simulink model "BEX7_CANOpen_Torque_Speed_Position_Control_Generic_2022b"  (R2022b)
settings: Solver=VariableStepAuto  StartTime=0.0  StopTime=inf  RelTol=1e-3
(part 2 of 2)

== system BEX7_CANOpen_Torque_Speed_Position_Control_Generic_2022b/Tx/Subsystem2/Enabled Subsystem1 ==
  CurrentLimit : Inport
  Enable : EnablePort
  Constant6 : Constant  Value=0  OutDataTypeStr=uint8
  SetCurrentLimit : Subsystem
  Result : Outport
  Error : Outport  Port=2
  wires:
  Constant6/1 -> SetCurrentLimit/1(Address)
  CurrentLimit/1 -> SetCurrentLimit/2(Value)
  SetCurrentLimit/2(Error) -> Error/1
  SetCurrentLimit/1(Result) -> Result/1

== system BEX7_CANOpen_Torque_Speed_Position_Control_Generic_2022b/Tx/Subsystem2/Enabled Subsystem2 ==
  Number of Poles : Inport
  Enable : EnablePort
  Constant6 : Constant  Value=0  OutDataTypeStr=uint8
  SetMotorPoleCounts : Subsystem
  Result : Outport
  Error : Outport  Port=2
  wires:
  Number of Poles/1 -> SetMotorPoleCounts/2(Value)
  Constant6/1 -> SetMotorPoleCounts/1(Address)
  SetMotorPoleCounts/2(Error) -> Error/1
  SetMotorPoleCounts/1(Result) -> Result/1

== system BEX7_CANOpen_Torque_Speed_Position_Control_Generic_2022b/Tx/Subsystem2/Enabled Subsystem3 ==
  EncoderLines : Inport
  Enable : EnablePort
  Constant6 : Constant  Value=0  OutDataTypeStr=uint8
  SetEncoderLines : Subsystem
  Result : Outport
  Error : Outport  Port=2
  wires:
  Constant6/1 -> SetEncoderLines/1(Address)
  EncoderLines/1 -> SetEncoderLines/2(Value)
  SetEncoderLines/2(Error) -> Error/1
  SetEncoderLines/1(Result) -> Result/1

== system BEX7_CANOpen_Torque_Speed_Position_Control_Generic_2022b/Tx/Subsystem2/Enabled Subsystem4 ==
  C.C.W Offset : Inport
  Enable : EnablePort
  Constant6 : Constant  Value=0  OutDataTypeStr=uint8
  SetEncoderHallCcwOffset : Subsystem
  Result : Outport
  Error : Outport  Port=2
  wires:
  C.C.W Offset/1 -> SetEncoderHallCcwOffset/2(Value)
  Constant6/1 -> SetEncoderHallCcwOffset/1(Address)
  SetEncoderHallCcwOffset/2(Error) -> Error/1
  SetEncoderHallCcwOffset/1(Result) -> Result/1

== system BEX7_CANOpen_Torque_Speed_Position_Control_Generic_2022b/Tx/Subsystem2/Enabled Subsystem5 ==
  C.W Offset : Inport
  Enable : EnablePort
  Constant6 : Constant  Value=0  OutDataTypeStr=uint8
  SetEncoderHallCwOffset : Subsystem
  Result : Outport
  Error : Outport  Port=2
  wires:
  Constant6/1 -> SetEncoderHallCwOffset/1(Address)
  C.W Offset/1 -> SetEncoderHallCwOffset/2(Value)
  SetEncoderHallCwOffset/2(Error) -> Error/1
  SetEncoderHallCwOffset/1(Result) -> Result/1

== system BEX7_CANOpen_Torque_Speed_Position_Control_Generic_2022b/Tx/Subsystem2/Enabled Subsystem6 ==
  SpeedLimit : Inport
  Enable : EnablePort
  Constant6 : Constant  Value=0  OutDataTypeStr=uint8
  SetSpeedLimit : Subsystem
  Result : Outport
  Error : Outport  Port=2
  wires:
  SpeedLimit/1 -> SetSpeedLimit/2(Value)
  Constant6/1 -> SetSpeedLimit/1(Address)
  SetSpeedLimit/2(Error) -> Error/1
  SetSpeedLimit/1(Result) -> Result/1

== system BEX7_CANOpen_Torque_Speed_Position_Control_Generic_2022b/Tx/Subsystem2/Enabled Subsystem7 ==
  ControlMode : Inport
  Enable : EnablePort
  Constant6 : Constant  Value=0  OutDataTypeStr=uint8
  SetControlMode : Subsystem
  Result : Outport
  Error : Outport  Port=2
  wires:
  Constant6/1 -> SetControlMode/1(Address)
  ControlMode/1 -> SetControlMode/2(Value)
  SetControlMode/2(Error) -> Error/1
  SetControlMode/1(Result) -> Result/1

== system BEX7_CANOpen_Torque_Speed_Position_Control_Generic_2022b/Tx/Subsystem2/Enabled Subsystem8 ==
  MotorType : Inport
  Enable : EnablePort
  Constant6 : Constant  Value=0  OutDataTypeStr=uint8
  SetMotorType : Subsystem
  Result : Outport
  Error : Outport  Port=2
  wires:
  MotorType/1 -> SetMotorType/2(Value)
  Constant6/1 -> SetMotorType/1(Address)
  SetMotorType/2(Error) -> Error/1
  SetMotorType/1(Result) -> Result/1

== system BEX7_CANOpen_Torque_Speed_Position_Control_Generic_2022b/Tx/Subsystem2/Enabled Subsystem9 ==
  FeedbackMode : Inport
  Enable : EnablePort
  Constant6 : Constant  Value=0  OutDataTypeStr=uint8
  SetFeedBackControlMode : Subsystem
  Result : Outport
  Error : Outport  Port=2
  wires:
  Constant6/1 -> SetFeedBackControlMode/1(Address)
  FeedbackMode/1 -> SetFeedBackControlMode/2(Value)
  SetFeedBackControlMode/2(Error) -> Error/1
  SetFeedBackControlMode/1(Result) -> Result/1

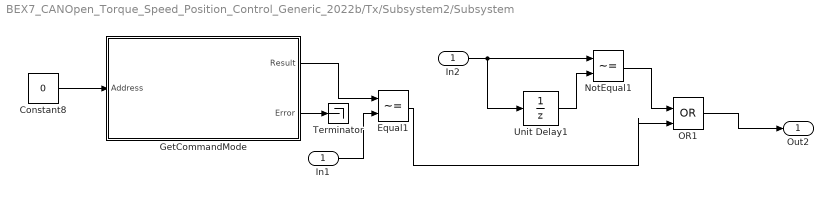
== system BEX7_CANOpen_Torque_Speed_Position_Control_Generic_2022b/Tx/Subsystem2/Subsystem ==
  In1 : Inport
  Constant8 : Constant  Value=0  OutDataTypeStr=uint8
  Equal1 : RelationalOperator  Operator=~=  OutDataTypeStr=boolean  RndMeth=Simplest  InputSameDT=off
  GetCommandMode : Subsystem
  In2 : InportShadow
  NotEqual1 : RelationalOperator  Operator=~=  OutDataTypeStr=boolean  RndMeth=Simplest  InputSameDT=off
  OR1 : Logic  Operator=OR  IconShape=distinctive  AllPortsSameDT=off  OutDataTypeStr=boolean
  Terminator : Terminator
  Unit Delay1 : UnitDelay  InitialCondition=2.1651  SampleTime=-1  HasFrameUpgradeWarning=on
  Out2 : Outport
  wires:
  In2/1 -> Unit Delay1/1, NotEqual1/1
  In1/1 -> Equal1/2
  GetCommandMode/2(Error) -> Terminator/1
  Equal1/1 -> OR1/2
  NotEqual1/1 -> OR1/1
  GetCommandMode/1(Result) -> Equal1/1
  Constant8/1 -> GetCommandMode/1(Address)
  Unit Delay1/1 -> NotEqual1/2
  OR1/1 -> Out2/1

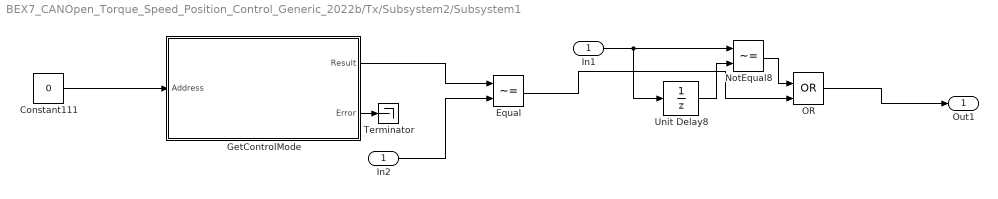
== system BEX7_CANOpen_Torque_Speed_Position_Control_Generic_2022b/Tx/Subsystem2/Subsystem1 ==
  In1 : Inport
  Constant111 : Constant  Value=0  OutDataTypeStr=uint8
  Equal : RelationalOperator  Operator=~=  OutDataTypeStr=boolean  RndMeth=Simplest  InputSameDT=off
  GetControlMode : Subsystem
  In2 : InportShadow
  NotEqual8 : RelationalOperator  Operator=~=  OutDataTypeStr=boolean  RndMeth=Simplest  InputSameDT=off
  OR : Logic  Operator=OR  IconShape=distinctive  AllPortsSameDT=off  OutDataTypeStr=boolean
  Terminator : Terminator
  Unit Delay8 : UnitDelay  InitialCondition=2.1651  SampleTime=-1  HasFrameUpgradeWarning=on
  Out1 : Outport
  wires:
  OR/1 -> Out1/1
  Unit Delay8/1 -> NotEqual8/2
  In1/1 -> Unit Delay8/1, NotEqual8/1
  Equal/1 -> OR/2
  GetControlMode/1(Result) -> Equal/1
  NotEqual8/1 -> OR/1
  GetControlMode/2(Error) -> Terminator/1
  Constant111/1 -> GetControlMode/1(Address)
  In2/1 -> Equal/2

== system BEX7_CANOpen_Torque_Speed_Position_Control_Generic_2022b/Tx/Subsystem1/Enabled Subsystem/SetTorqueReferenceIq ==
  Address : Inport  OutDataTypeStr=uint8  LockScale=on
  Value : Inport  Port=2  OutDataTypeStr=single  LockScale=on
  Display12 : Display
      settings: Format=decimal (Stored Integer)
  Display13 : Display
      settings: Format=decimal (Stored Integer)
  S-Function Builder4 : S-Function  Priority=2  FunctionName=SetTorqueReferenceIq  SFunctionModules=SetTorqueReferenceIq_wrapper  SFunctionDeploymentMode=off  EnableBusSupport=off  mask(S-Function Builder){}
      mask help: Simulink:masks:SFunctionBuilder_MD
      mask init: same as BEX7_CANOpen_Torque_Speed_Position_Control_Generic_2022b/Subsystem1/Subsystem/S-Function Builder1
      settings: CopyFcn=set_param(gcbh,'LinkStatus','none')  OpenFcn=sfunctionwizard(gcbh)
      mask Display: plot(val(:,1),val(:,2)),disp(sys),port_label('input',1,'Address'),port_label('input',2,'Value'),port_label('output',1,'Result'),port_label('output',2,'Error')
  Result : Outport  OutDataTypeStr=boolean
  Error : Outport  Port=2  OutDataTypeStr=int32
  wires:
  Address/1 -> S-Function Builder4/1
  S-Function Builder4/2 -> Error/1, Display13/1
  S-Function Builder4/1 -> Result/1, Display12/1
  Value/1 -> S-Function Builder4/2

== system BEX7_CANOpen_Torque_Speed_Position_Control_Generic_2022b/Tx/Subsystem1/Enabled Subsystem1/SpeedRef ==
  Address : Inport
  Value : Inport  Port=2
  Display16 : Display
      settings: Format=decimal (Stored Integer)
  Display17 : Display
      settings: Format=decimal (Stored Integer)
  S-Function Builder8 : S-Function  Priority=2  FunctionName=SetSpeedReference  SFunctionModules=SetSpeedReference_wrapper  SFunctionDeploymentMode=off  EnableBusSupport=off  mask(S-Function Builder){}
      mask help: Simulink:masks:SFunctionBuilder_MD
      mask init: same as BEX7_CANOpen_Torque_Speed_Position_Control_Generic_2022b/Subsystem1/Subsystem/S-Function Builder1
      settings: CopyFcn=set_param(gcbh,'LinkStatus','none')  OpenFcn=sfunctionwizard(gcbh)
      mask Display:
      | plot(val(:,1),val(:,2))
      | disp(sys)
      | port_label('input',1,'Address')
      | port_label('input',2,'Value')
      | port_label('output',1,'Result')
      | port_label('output',2,'Error')
  Result : Outport
  Error : Outport  Port=2
  wires:
  Address/1 -> S-Function Builder8/1
  S-Function Builder8/1 -> Result/1, Display16/1
  S-Function Builder8/2 -> Error/1, Display17/1
  Value/1 -> S-Function Builder8/2

== system BEX7_CANOpen_Torque_Speed_Position_Control_Generic_2022b/Tx/Subsystem1/Enabled Subsystem10/EmergencyStop1 ==
  note: Error
  Address : Inport
  Display22 : Display
      settings: Format=decimal (Stored Integer)
  Display23 : Display
      settings: Format=decimal (Stored Integer)
  S-Function Builder11 : S-Function  Priority=2  FunctionName=EmergencyStop  SFunctionModules=EmergencyStop_wrapper  SFunctionDeploymentMode=off  EnableBusSupport=off  mask(S-Function Builder){}
      mask help: Simulink:masks:SFunctionBuilder_MD
      mask init: same as BEX7_CANOpen_Torque_Speed_Position_Control_Generic_2022b/Subsystem1/Subsystem/S-Function Builder1
      settings: CopyFcn=set_param(gcbh,'LinkStatus','none')  OpenFcn=sfunctionwizard(gcbh)
      mask Display:
      | plot(val(:,1),val(:,2))
      | disp(sys)
      | port_label('input',1,'Address')
      | port_label('output',1,'Result')
      | port_label('output',2,'Error')
  Result : Outport
  Error : Outport  Port=2
  wires:
  S-Function Builder11/2 -> Error/1, Display23/1
  S-Function Builder11/1 -> Result/1, Display22/1
  Address/1 -> S-Function Builder11/1

== system BEX7_CANOpen_Torque_Speed_Position_Control_Generic_2022b/Tx/Subsystem1/Enabled Subsystem2/SetPositionRef ==
  Address : Inport
  Value : Inport  Port=2
  S-Function Builder30 : S-Function  Priority=2  FunctionName=SetPositionReference  SFunctionModules=SetPositionReference_wrapper  SFunctionDeploymentMode=off  EnableBusSupport=off  mask(S-Function Builder){}
      mask help: Simulink:masks:SFunctionBuilder_MD
      mask init: same as BEX7_CANOpen_Torque_Speed_Position_Control_Generic_2022b/Subsystem1/Subsystem/S-Function Builder1
      settings: CopyFcn=set_param(gcbh,'LinkStatus','none')  OpenFcn=sfunctionwizard(gcbh)
      mask Display:
      | plot(val(:,1),val(:,2))
      | disp(sys)
      | port_label('input',1,'Address')
      | port_label('input',2,'Value')
      | port_label('output',1,'Result')
      | port_label('output',2,'Error')
  Result : Outport
  Error : Outport  Port=2
  wires:
  S-Function Builder30/1 -> Result/1
  S-Function Builder30/2 -> Error/1
  Value/1 -> S-Function Builder30/2
  Address/1 -> S-Function Builder30/1

== system BEX7_CANOpen_Torque_Speed_Position_Control_Generic_2022b/Tx/Subsystem1/Enabled Subsystem3/SetMotorDirection ==
  Address : Inport
  Value : Inport  Port=2
  S-Function Builder15 : S-Function  Priority=2  FunctionName=SetMotorDirection  SFunctionModules=SetMotorDirection_wrapper  SFunctionDeploymentMode=off  EnableBusSupport=off  mask(S-Function Builder){}
      mask help: Simulink:masks:SFunctionBuilder_MD
      mask init: same as BEX7_CANOpen_Torque_Speed_Position_Control_Generic_2022b/Subsystem1/Subsystem/S-Function Builder1
      settings: CopyFcn=set_param(gcbh,'LinkStatus','none')  OpenFcn=sfunctionwizard(gcbh)
      mask Display: plot(val(:,1),val(:,2)),disp(sys),port_label('input',1,'Address'),port_label('input',2,'Value'),port_label('output',1,'Result'),port_label('output',2,'Error')
  Result : Outport
  Error : Outport  Port=2
  wires:
  S-Function Builder15/2 -> Error/1
  Value/1 -> S-Function Builder15/2
  S-Function Builder15/1 -> Result/1
  Address/1 -> S-Function Builder15/1

== system BEX7_CANOpen_Torque_Speed_Position_Control_Generic_2022b/Tx/Subsystem1/Enabled Subsystem4/SetSpeed Kp ==
  Address : Inport
  Value : Inport  Port=2
  Display26 : Display
      settings: Format=decimal (Stored Integer)
  Display27 : Display
      settings: Format=decimal (Stored Integer)
  S-Function Builder13 : S-Function  Priority=2  FunctionName=SetSpeedControllerKp  SFunctionModules=SetSpeedControllerKp_wrapper  SFunctionDeploymentMode=off  EnableBusSupport=off  mask(S-Function Builder){}
      mask help: Simulink:masks:SFunctionBuilder_MD
      mask init: same as BEX7_CANOpen_Torque_Speed_Position_Control_Generic_2022b/Subsystem1/Subsystem/S-Function Builder1
      settings: CopyFcn=set_param(gcbh,'LinkStatus','none')  OpenFcn=sfunctionwizard(gcbh)
      mask Display:
      | plot(val(:,1),val(:,2))
      | disp(sys)
      | port_label('input',1,'Address')
      | port_label('input',2,'Value')
      | port_label('output',1,'Result')
      | port_label('output',2,'Error')
  Result : Outport
  Error : Outport  Port=2
  wires:
  S-Function Builder13/1 -> Result/1, Display26/1
  S-Function Builder13/2 -> Error/1, Display27/1
  Address/1 -> S-Function Builder13/1
  Value/1 -> S-Function Builder13/2

== system BEX7_CANOpen_Torque_Speed_Position_Control_Generic_2022b/Tx/Subsystem1/Enabled Subsystem5/SetSpeed Ki ==
  Address : Inport
  Value : Inport  Port=2
  Display28 : Display
      settings: Format=decimal (Stored Integer)
  Display29 : Display
      settings: Format=decimal (Stored Integer)
  S-Function Builder14 : S-Function  Priority=2  FunctionName=SetSpeedControllerKi  SFunctionModules=SetSpeedControllerKi_wrapper  SFunctionDeploymentMode=off  EnableBusSupport=off  mask(S-Function Builder){}
      mask help: Simulink:masks:SFunctionBuilder_MD
      mask init: same as BEX7_CANOpen_Torque_Speed_Position_Control_Generic_2022b/Subsystem1/Subsystem/S-Function Builder1
      settings: CopyFcn=set_param(gcbh,'LinkStatus','none')  OpenFcn=sfunctionwizard(gcbh)
      mask Display:
      | plot(val(:,1),val(:,2))
      | disp(sys)
      | port_label('input',1,'Address')
      | port_label('input',2,'Value')
      | port_label('output',1,'Result')
      | port_label('output',2,'Error')
  Result : Outport
  Error : Outport  Port=2
  wires:
  S-Function Builder14/1 -> Result/1, Display28/1
  Value/1 -> S-Function Builder14/2
  S-Function Builder14/2 -> Error/1, Display29/1
  Address/1 -> S-Function Builder14/1

== system BEX7_CANOpen_Torque_Speed_Position_Control_Generic_2022b/Tx/Subsystem1/Enabled Subsystem6/SetPositionControllerKp ==
  Address : Inport
  Value : Inport  Port=2
  Display62 : Display
      settings: Format=decimal (Stored Integer)
  Display63 : Display
      settings: Format=decimal (Stored Integer)
  S-Function Builder31 : S-Function  Priority=2  FunctionName=SetPositionControllerKp  SFunctionModules=SetPositionControllerKp_wrapper  SFunctionDeploymentMode=off  EnableBusSupport=off  mask(S-Function Builder){}
      mask help: Simulink:masks:SFunctionBuilder_MD
      mask init: same as BEX7_CANOpen_Torque_Speed_Position_Control_Generic_2022b/Subsystem1/Subsystem/S-Function Builder1
      settings: CopyFcn=set_param(gcbh,'LinkStatus','none')  OpenFcn=sfunctionwizard(gcbh)
      mask Display:
      | plot(val(:,1),val(:,2))
      | disp(sys)
      | port_label('input',1,'Address')
      | port_label('input',2,'Value')
      | port_label('output',1,'Result')
      | port_label('output',2,'Error')
  Result : Outport
  Error : Outport  Port=2
  wires:
  S-Function Builder31/2 -> Error/1, Display63/1
  Value/1 -> S-Function Builder31/2
  Address/1 -> S-Function Builder31/1
  S-Function Builder31/1 -> Result/1, Display62/1

== system BEX7_CANOpen_Torque_Speed_Position_Control_Generic_2022b/Tx/Subsystem1/Enabled Subsystem7/SetPositionControllerKi ==
  Address : Inport
  Value : Inport  Port=2
  Display64 : Display
      settings: Format=decimal (Stored Integer)
  Display65 : Display
      settings: Format=decimal (Stored Integer)
  S-Function Builder32 : S-Function  Priority=2  FunctionName=SetPositionControllerKi  SFunctionModules=SetPositionControllerKi_wrapper  SFunctionDeploymentMode=off  EnableBusSupport=off  mask(S-Function Builder){}
      mask help: Simulink:masks:SFunctionBuilder_MD
      mask init: same as BEX7_CANOpen_Torque_Speed_Position_Control_Generic_2022b/Subsystem1/Subsystem/S-Function Builder1
      settings: CopyFcn=set_param(gcbh,'LinkStatus','none')  OpenFcn=sfunctionwizard(gcbh)
      mask Display:
      | plot(val(:,1),val(:,2))
      | disp(sys)
      | port_label('input',1,'Address')
      | port_label('input',2,'Value')
      | port_label('output',1,'Result')
      | port_label('output',2,'Error')
  Result : Outport
  Error : Outport  Port=2
  wires:
  S-Function Builder32/1 -> Result/1, Display64/1
  Value/1 -> S-Function Builder32/2
  S-Function Builder32/2 -> Error/1, Display65/1
  Address/1 -> S-Function Builder32/1

== system BEX7_CANOpen_Torque_Speed_Position_Control_Generic_2022b/Tx/Subsystem1/Enabled Subsystem8/SetCurrentControlKp ==
  Address : Inport
  Value : Inport  Port=2
  Display52 : Display
      settings: Format=decimal (Stored Integer)
  Display53 : Display
      settings: Format=decimal (Stored Integer)
  S-Function Builder26 : S-Function  Priority=2  FunctionName=SetCurrentControllerKp  SFunctionModules=SetCurrentControllerKp_wrapper  SFunctionDeploymentMode=off  EnableBusSupport=off  mask(S-Function Builder){}
      mask help: Simulink:masks:SFunctionBuilder_MD
      mask init: same as BEX7_CANOpen_Torque_Speed_Position_Control_Generic_2022b/Subsystem1/Subsystem/S-Function Builder1
      settings: CopyFcn=set_param(gcbh,'LinkStatus','none')  OpenFcn=sfunctionwizard(gcbh)
      mask Display:
      | plot(val(:,1),val(:,2))
      | disp(sys)
      | port_label('input',1,'Address')
      | port_label('input',2,'Value')
      | port_label('output',1,'Result')
      | port_label('output',2,'Error')
  Result : Outport
  Error : Outport  Port=2
  wires:
  Value/1 -> S-Function Builder26/2
  S-Function Builder26/1 -> Result/1, Display52/1
  Address/1 -> S-Function Builder26/1
  S-Function Builder26/2 -> Error/1, Display53/1

== system BEX7_CANOpen_Torque_Speed_Position_Control_Generic_2022b/Tx/Subsystem1/Enabled Subsystem9/SetCurrentControlKi ==
  Address : Inport
  Value : Inport  Port=2
  Display54 : Display
      settings: Format=decimal (Stored Integer)
  Display55 : Display
      settings: Format=decimal (Stored Integer)
  S-Function Builder27 : S-Function  Priority=2  FunctionName=SetCurrentControllerKi  SFunctionModules=SetCurrentControllerKi_wrapper  SFunctionDeploymentMode=off  EnableBusSupport=off  mask(S-Function Builder){}
      mask help: Simulink:masks:SFunctionBuilder_MD
      mask init: same as BEX7_CANOpen_Torque_Speed_Position_Control_Generic_2022b/Subsystem1/Subsystem/S-Function Builder1
      settings: CopyFcn=set_param(gcbh,'LinkStatus','none')  OpenFcn=sfunctionwizard(gcbh)
      mask Display:
      | plot(val(:,1),val(:,2))
      | disp(sys)
      | port_label('input',1,'Address')
      | port_label('input',2,'Value')
      | port_label('output',1,'Result')
      | port_label('output',2,'Error')
  Result : Outport
  Error : Outport  Port=2
  wires:
  Value/1 -> S-Function Builder27/2
  S-Function Builder27/1 -> Result/1, Display54/1
  S-Function Builder27/2 -> Error/1, Display55/1
  Address/1 -> S-Function Builder27/1

== system BEX7_CANOpen_Torque_Speed_Position_Control_Generic_2022b/Tx/Subsystem1/Subsystem/GetMotorDirection ==
  Address : Inport
  S-Function Builder82 : S-Function  Priority=3  FunctionName=GetMotorDirection  SFunctionModules=GetMotorDirection_wrapper  SFunctionDeploymentMode=off  EnableBusSupport=off  mask(S-Function Builder){}
      mask help: Simulink:masks:SFunctionBuilder_MD
      mask init: same as BEX7_CANOpen_Torque_Speed_Position_Control_Generic_2022b/Subsystem1/Subsystem/S-Function Builder1
      settings: CopyFcn=set_param(gcbh,'LinkStatus','none')  OpenFcn=sfunctionwizard(gcbh)
      mask Display:
      | plot(val(:,1),val(:,2))
      | disp(sys)
      | port_label('input',1,'Address')
      | port_label('output',1,'Result')
      | port_label('output',2,'Error')
  Result : Outport
  Error : Outport  Port=2
  wires:
  S-Function Builder82/2 -> Error/1
  S-Function Builder82/1 -> Result/1
  Address/1 -> S-Function Builder82/1

== system BEX7_CANOpen_Torque_Speed_Position_Control_Generic_2022b/Tx/Subsystem2/Enabled Subsystem/SetCommandMode ==
  Address : Inport  OutDataTypeStr=uint8  LockScale=on
  Value : Inport  Port=2  OutDataTypeStr=boolean  LockScale=on
  S-Function Builder2 : S-Function  Priority=2  FunctionName=SetCommandMode  SFunctionModules=SetCommandMode_wrapper  SFunctionDeploymentMode=off  EnableBusSupport=off  mask(S-Function Builder){}
      mask help: Simulink:masks:SFunctionBuilder_MD
      mask init: same as BEX7_CANOpen_Torque_Speed_Position_Control_Generic_2022b/Subsystem1/Subsystem/S-Function Builder1
      settings: CopyFcn=set_param(gcbh,'LinkStatus','none')  OpenFcn=sfunctionwizard(gcbh)
      mask Display: plot(val(:,1),val(:,2)),disp(sys),port_label('input',1,'Address'),port_label('input',2,'Value'),port_label('output',1,'Result'),port_label('output',2,'Error')
  Result : Outport  OutDataTypeStr=boolean
  Error : Outport  Port=2
  wires:
  S-Function Builder2/1 -> Result/1
  S-Function Builder2/2 -> Error/1
  Address/1 -> S-Function Builder2/1
  Value/1 -> S-Function Builder2/2

== system BEX7_CANOpen_Torque_Speed_Position_Control_Generic_2022b/Tx/Subsystem2/Enabled Subsystem1/SetCurrentLimit ==
  Address : Inport  Tag=Address  LockScale=on
  Value : Inport  Port=2  LockScale=on
  Display1 : Display
      settings: Format=decimal (Stored Integer)
  Display10 : Display
      settings: Format=decimal (Stored Integer)
  S-Function Builder : S-Function  Priority=2  FunctionName=SetCurrentLimit  SFunctionModules=SetCurrentLimit_wrapper  SFunctionDeploymentMode=off  EnableBusSupport=off  mask(S-Function Builder){}
      mask help: Simulink:masks:SFunctionBuilder_MD
      mask init: same as BEX7_CANOpen_Torque_Speed_Position_Control_Generic_2022b/Subsystem1/Subsystem/S-Function Builder1
      settings: CopyFcn=set_param(gcbh,'LinkStatus','none')  OpenFcn=sfunctionwizard(gcbh)
      mask Display: plot(val(:,1),val(:,2)),disp(sys),port_label('input',1,'Address'),port_label('input',2,'Value'),port_label('output',1,'Result'),port_label('output',2,'Error')
  Result : Outport  OutDataTypeStr=boolean
  Error : Outport  Port=2  OutDataTypeStr=int32
  wires:
  Value/1 -> S-Function Builder/2
  S-Function Builder/2 -> Error/1, Display10/1
  S-Function Builder/1 -> Result/1, Display1/1
  Address/1 -> S-Function Builder/1

== system BEX7_CANOpen_Torque_Speed_Position_Control_Generic_2022b/Tx/Subsystem2/Enabled Subsystem2/SetMotorPoleCounts ==
  Address : Inport
  Value : Inport  Port=2
  Display36 : Display
      settings: Format=decimal (Stored Integer)
  Display37 : Display
      settings: Format=decimal (Stored Integer)
  S-Function Builder18 : S-Function  Priority=2  FunctionName=SetMotorPolesCounts  SFunctionModules=SetMotorPolesCounts_wrapper  SFunctionDeploymentMode=off  EnableBusSupport=off  mask(S-Function Builder){}
      mask help: Simulink:masks:SFunctionBuilder_MD
      mask init: same as BEX7_CANOpen_Torque_Speed_Position_Control_Generic_2022b/Subsystem1/Subsystem/S-Function Builder1
      settings: CopyFcn=set_param(gcbh,'LinkStatus','none')  OpenFcn=sfunctionwizard(gcbh)
      mask Display:
      | plot(val(:,1),val(:,2))
      | disp(sys)
      | port_label('input',1,'Address')
      | port_label('input',2,'Value')
      | port_label('output',1,'Result')
      | port_label('output',2,'Error')
  Result : Outport
  Error : Outport  Port=2
  wires:
  S-Function Builder18/1 -> Result/1, Display36/1
  Value/1 -> S-Function Builder18/2
  S-Function Builder18/2 -> Error/1, Display37/1
  Address/1 -> S-Function Builder18/1

== system BEX7_CANOpen_Torque_Speed_Position_Control_Generic_2022b/Tx/Subsystem2/Enabled Subsystem3/SetEncoderLines ==
  Address : Inport
  Value : Inport  Port=2
  Display38 : Display
      settings: Format=decimal (Stored Integer)
  Display39 : Display
      settings: Format=decimal (Stored Integer)
  S-Function Builder19 : S-Function  Priority=2  FunctionName=SetIncrementalEncoderLines  SFunctionModules=SetIncrementalEncoderLines_wrapper  SFunctionDeploymentMode=off  EnableBusSupport=off  mask(S-Function Builder){}
      mask help: Simulink:masks:SFunctionBuilder_MD
      mask init: same as BEX7_CANOpen_Torque_Speed_Position_Control_Generic_2022b/Subsystem1/Subsystem/S-Function Builder1
      settings: CopyFcn=set_param(gcbh,'LinkStatus','none')  OpenFcn=sfunctionwizard(gcbh)
      mask Display:
      | plot(val(:,1),val(:,2))
      | disp(sys)
      | port_label('input',1,'Address')
      | port_label('input',2,'Value')
      | port_label('output',1,'Result')
      | port_label('output',2,'Error')
  Result : Outport
  Error : Outport  Port=2
  wires:
  S-Function Builder19/1 -> Result/1, Display38/1
  Value/1 -> S-Function Builder19/2
  S-Function Builder19/2 -> Error/1, Display39/1
  Address/1 -> S-Function Builder19/1

== system BEX7_CANOpen_Torque_Speed_Position_Control_Generic_2022b/Tx/Subsystem2/Enabled Subsystem4/SetEncoderHallCcwOffset ==
  Address : Inport
  Value : Inport  Port=2
  Display84 : Display
      settings: Format=decimal (Stored Integer)
  Display85 : Display
      settings: Format=decimal (Stored Integer)
  S-Function Builder42 : S-Function  Priority=2  FunctionName=SetEncoderHallCcwOffset  SFunctionModules=SetEncoderHallCcwOffset_wrapper  SFunctionDeploymentMode=off  EnableBusSupport=off  mask(S-Function Builder){}
      mask help: Simulink:masks:SFunctionBuilder_MD
      mask init: same as BEX7_CANOpen_Torque_Speed_Position_Control_Generic_2022b/Subsystem1/Subsystem/S-Function Builder1
      settings: CopyFcn=set_param(gcbh,'LinkStatus','none')  OpenFcn=sfunctionwizard(gcbh)
      mask Display: plot(val(:,1),val(:,2)),disp(sys),port_label('input',1,'Address'),port_label('input',2,'Value'),port_label('output',1,'Result'),port_label('output',2,'Error')
  Result : Outport
  Error : Outport  Port=2
  wires:
  S-Function Builder42/2 -> Error/1, Display85/1
  Value/1 -> S-Function Builder42/2
  S-Function Builder42/1 -> Result/1, Display84/1
  Address/1 -> S-Function Builder42/1

== system BEX7_CANOpen_Torque_Speed_Position_Control_Generic_2022b/Tx/Subsystem2/Enabled Subsystem5/SetEncoderHallCwOffset ==
  Address : Inport
  Value : Inport  Port=2
  S-Function Builder43 : S-Function  Priority=2  FunctionName=SetEncoderHallCwOffset  SFunctionModules=SetEncoderHallCwOffset_wrapper  SFunctionDeploymentMode=off  EnableBusSupport=off  mask(S-Function Builder){}
      mask help: Simulink:masks:SFunctionBuilder_MD
      mask init: same as BEX7_CANOpen_Torque_Speed_Position_Control_Generic_2022b/Subsystem1/Subsystem/S-Function Builder1
      settings: CopyFcn=set_param(gcbh,'LinkStatus','none')  OpenFcn=sfunctionwizard(gcbh)
      mask Display:
      | plot(val(:,1),val(:,2))
      | disp(sys)
      | port_label('input',1,'Address')
      | port_label('input',2,'Value')
      | port_label('output',1,'Result')
      | port_label('output',2,'Error')
  Result : Outport
  Error : Outport  Port=2
  wires:
  Address/1 -> S-Function Builder43/1
  S-Function Builder43/2 -> Error/1
  S-Function Builder43/1 -> Result/1
  Value/1 -> S-Function Builder43/2

== system BEX7_CANOpen_Torque_Speed_Position_Control_Generic_2022b/Tx/Subsystem2/Enabled Subsystem6/SetSpeedLimit ==
  Address : Inport
  Value : Inport  Port=2
  Display40 : Display
      settings: Format=decimal (Stored Integer)
  Display41 : Display
      settings: Format=decimal (Stored Integer)
  S-Function Builder20 : S-Function  Priority=2  FunctionName=SetSpeedLimit  SFunctionModules=SetSpeedLimit_wrapper  SFunctionDeploymentMode=off  EnableBusSupport=off  mask(S-Function Builder){}
      mask help: Simulink:masks:SFunctionBuilder_MD
      mask init: same as BEX7_CANOpen_Torque_Speed_Position_Control_Generic_2022b/Subsystem1/Subsystem/S-Function Builder1
      settings: CopyFcn=set_param(gcbh,'LinkStatus','none')  OpenFcn=sfunctionwizard(gcbh)
      mask Display:
      | plot(val(:,1),val(:,2))
      | disp(sys)
      | port_label('input',1,'Address')
      | port_label('input',2,'Value')
      | port_label('output',1,'Result')
      | port_label('output',2,'Error')
  Result : Outport
  Error : Outport  Port=2
  wires:
  Value/1 -> S-Function Builder20/2
  S-Function Builder20/1 -> Result/1, Display40/1
  S-Function Builder20/2 -> Error/1, Display41/1
  Address/1 -> S-Function Builder20/1

== system BEX7_CANOpen_Torque_Speed_Position_Control_Generic_2022b/Tx/Subsystem2/Enabled Subsystem7/SetControlMode ==
  Address : Inport
  Value : Inport  Port=2
  S-Function Builder25 : S-Function  Priority=2  FunctionName=SetControlMode  SFunctionModules=SetControlMode_wrapper  SFunctionDeploymentMode=off  EnableBusSupport=off  mask(S-Function Builder){}
      mask help: Simulink:masks:SFunctionBuilder_MD
      mask init: same as BEX7_CANOpen_Torque_Speed_Position_Control_Generic_2022b/Subsystem1/Subsystem/S-Function Builder1
      settings: CopyFcn=set_param(gcbh,'LinkStatus','none')  OpenFcn=sfunctionwizard(gcbh)
      mask Display: plot(val(:,1),val(:,2)),disp(sys),port_label('input',1,'Address'),port_label('input',2,'Value'),port_label('output',1,'Result'),port_label('output',2,'Error')
  Result : Outport
  Error : Outport  Port=2
  wires:
  S-Function Builder25/1 -> Result/1
  S-Function Builder25/2 -> Error/1
  Value/1 -> S-Function Builder25/2
  Address/1 -> S-Function Builder25/1

== system BEX7_CANOpen_Torque_Speed_Position_Control_Generic_2022b/Tx/Subsystem2/Enabled Subsystem8/SetMotorType ==
  Address : Inport
  Value : Inport  Port=2
  Display46 : Display
      settings: Format=decimal (Stored Integer)
  Display47 : Display
      settings: Format=decimal (Stored Integer)
  S-Function Builder23 : S-Function  Priority=2  FunctionName=SetMotorType  SFunctionModules=SetMotorType_wrapper  SFunctionDeploymentMode=off  EnableBusSupport=off  mask(S-Function Builder){}
      mask help: Simulink:masks:SFunctionBuilder_MD
      mask init: same as BEX7_CANOpen_Torque_Speed_Position_Control_Generic_2022b/Subsystem1/Subsystem/S-Function Builder1
      settings: CopyFcn=set_param(gcbh,'LinkStatus','none')  OpenFcn=sfunctionwizard(gcbh)
      mask Display:
      | plot(val(:,1),val(:,2))
      | disp(sys)
      | port_label('input',1,'Address')
      | port_label('input',2,'Value')
      | port_label('output',1,'Result')
      | port_label('output',2,'Error')
  Result : Outport
  Error : Outport  Port=2
  wires:
  S-Function Builder23/1 -> Result/1, Display46/1
  Value/1 -> S-Function Builder23/2
  S-Function Builder23/2 -> Error/1, Display47/1
  Address/1 -> S-Function Builder23/1

== system BEX7_CANOpen_Torque_Speed_Position_Control_Generic_2022b/Tx/Subsystem2/Enabled Subsystem9/SetFeedBackControlMode ==
  Address : Inport
  Value : Inport  Port=2
  S-Function Builder21 : S-Function  Priority=2  FunctionName=SetFeedbackControlMode  SFunctionModules=SetFeedbackControlMode_wrapper  SFunctionDeploymentMode=off  EnableBusSupport=off  mask(S-Function Builder){}
      mask help: Simulink:masks:SFunctionBuilder_MD
      mask init: same as BEX7_CANOpen_Torque_Speed_Position_Control_Generic_2022b/Subsystem1/Subsystem/S-Function Builder1
      settings: CopyFcn=set_param(gcbh,'LinkStatus','none')  OpenFcn=sfunctionwizard(gcbh)
      mask Display:
      | plot(val(:,1),val(:,2))
      | disp(sys)
      | port_label('input',1,'Address')
      | port_label('input',2,'Value')
      | port_label('output',1,'Result')
      | port_label('output',2,'Error')
  Result : Outport
  Error : Outport  Port=2
  wires:
  S-Function Builder21/1 -> Result/1
  S-Function Builder21/2 -> Error/1
  Value/1 -> S-Function Builder21/2
  Address/1 -> S-Function Builder21/1

== system BEX7_CANOpen_Torque_Speed_Position_Control_Generic_2022b/Tx/Subsystem2/Subsystem/GetCommandMode ==
  Address : Inport
  S-Function Builder3 : S-Function  Priority=3  FunctionName=GetCommandMode  SFunctionModules=GetCommandMode_wrapper  SFunctionDeploymentMode=off  EnableBusSupport=off  mask(S-Function Builder){}
      mask help: Simulink:masks:SFunctionBuilder_MD
      mask init: same as BEX7_CANOpen_Torque_Speed_Position_Control_Generic_2022b/Subsystem1/Subsystem/S-Function Builder1
      settings: CopyFcn=set_param(gcbh,'LinkStatus','none')  OpenFcn=sfunctionwizard(gcbh)
      mask Display:
      | plot(val(:,1),val(:,2))
      | disp(sys)
      | port_label('input',1,'Address')
      | port_label('output',1,'Result')
      | port_label('output',2,'Error')
  Result : Outport
  Error : Outport  Port=2
  wires:
  S-Function Builder3/2 -> Error/1
  S-Function Builder3/1 -> Result/1
  Address/1 -> S-Function Builder3/1

== system BEX7_CANOpen_Torque_Speed_Position_Control_Generic_2022b/Tx/Subsystem2/Subsystem1/GetControlMode ==
  Address : Inport
  S-Function Builder69 : S-Function  Priority=3  FunctionName=GetControlMode  SFunctionModules=GetControlMode_wrapper  SFunctionDeploymentMode=off  EnableBusSupport=off  mask(S-Function Builder){}
      mask help: Simulink:masks:SFunctionBuilder_MD
      mask init: same as BEX7_CANOpen_Torque_Speed_Position_Control_Generic_2022b/Subsystem1/Subsystem/S-Function Builder1
      settings: CopyFcn=set_param(gcbh,'LinkStatus','none')  OpenFcn=sfunctionwizard(gcbh)
      mask Display: plot(val(:,1),val(:,2)),disp(sys),port_label('input',1,'Address'),port_label('output',1,'Result'),port_label('output',2,'Error')
  Result : Outport
  Error : Outport  Port=2
  wires:
  Address/1 -> S-Function Builder69/1
  S-Function Builder69/1 -> Result/1
  S-Function Builder69/2 -> Error/1
